simulink model "PID_AutoTuning_tester"  (R2024b)
settings: Solver=FixedStepDiscrete  StartTime=0.0  StopTime=SimEndTime  FixedStep=TimeStep  RelTol=1e-3
undefined symbols (not defined in the file): ctrl_start_time, deadzone_comp_flag, deadzone_comp_val, I_gain_init, P_gain_init, TimeStep
libraries: slctrl_autotuning x1, slpidlib x1, SignalEditorBlockLib x1
settings Model: DataDictionary=system_data.sldd  Creator=tshintai  LastModifiedBy=tshintai
settings SolverCC: AlgebraicLoopSolver=TrustRegion
settings DataIOCC: SaveOutput=off  SaveTime=off
settings OptimizationCC: ReuseModelBlockBuffer=off
settings DebuggingCC: UnconnectedInputMsg=warning  UnconnectedOutputMsg=warning  UnconnectedLineMsg=warning
settings ModelReferenceCC: EnableRefExpFcnMdlSchedulingChecks=on
settings RTWCC: GPUComputeCapability=3.5  DLArmComputeVersion=19.05

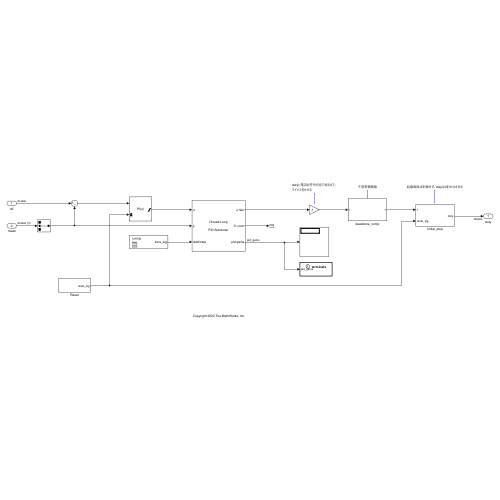
[thumbnail: Simulink's stored preview of the top-level diagram]
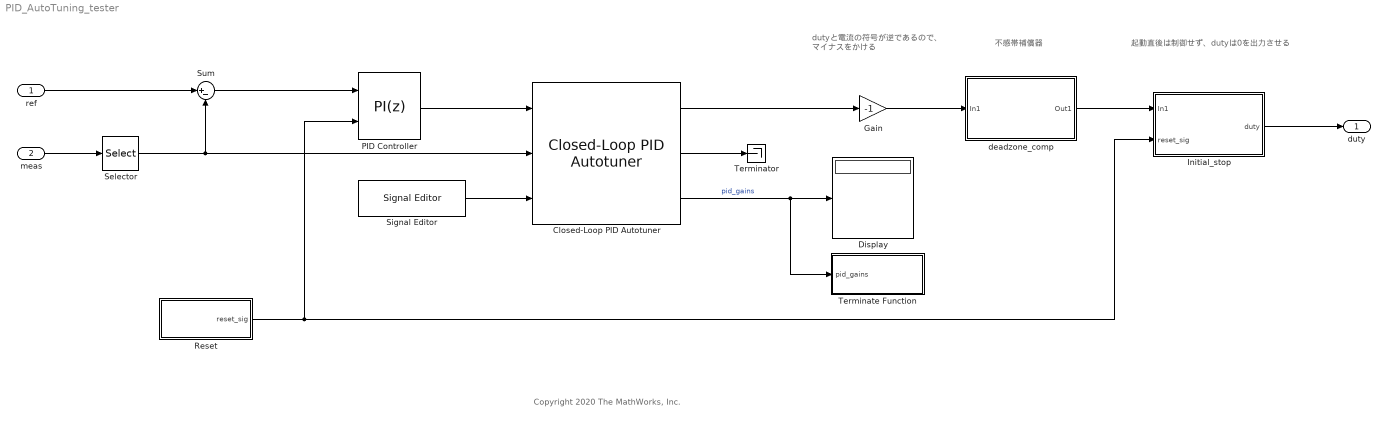
== system PID_AutoTuning_tester ==
  note: Copyright 2020 The MathWorks, Inc.
  note: dutyと電流の符号が逆であるので、
      | マイナスをかける
  note: 起動直後は制御せず、dutyは0を出力させる
  note: 不感帯補償器
  ref : Inport  OutDataTypeStr=double  PortDimensions=1  SampleTime=[0.0001,0]
  meas : Inport  Port=2  OutDataTypeStr=double  PortDimensions=3  SampleTime=[0.0001,0]
  Closed-Loop PID Autotuner : slctrl_autotuning/Closed-Loop PID Autotuner  PIDType=PI  PIDForm=Parallel  TimeDomain=discrete-time  DiscreteTs=TimeStep  TuningTs=0.2  UseTuningTs=off  IntegratorFormula=Forward Euler  FilterFormula=Forward Euler  ContinuousTs=0.02  Bandwidth=2000  UseExternalWC=off  TargetPM=60  UseExternalPM=off  UseExternalAchievedPM=off  ExperimentMode=Superposition  PlantType=Integrating  PlantSign=Positive  AmpSine=0.05  UseExternalAmpSine=off  UseExternalFRD=off  UseExternalU0=off  UseCompanion=off  NotDeployTuningModule=off  UsePLCCoder=off  OutputMode=control action + perturbation  BlockDataType=double  UseConnectedPID=on  blockpath=[]  tunedP=0  tunedI=0  tunedD=0  tunedN=100  tunedPM=0  EstimationWindowSize=3  UseExternalTuningParams=off  SingleMultiRateVariant=SingleSamplingRate  NumEstimationPeriods=4  NumSettlingPeriods=2  NumOfPRBSPeriod=1  PRBSSignalOrder=12  ExperimentModeVariant=VariantSuperimposed  OutputChoice=VariantCandD  ConvergenceCalcVariant=ConvSuperpositionPRBSVariant
  Display : Display
  Gain : Gain  Gain=-1
  Initial_stop : Subsystem
  PID Controller : slpidlib/PID Controller  Controller=PI  Form=Parallel  TimeDomain=Discrete-time  UseExternalTs=off  SampleTime=-1  IntegratorMethod=Forward Euler  FilterMethod=Forward Euler  ControllerParametersSource=internal  P=P_gain_init  I=I_gain_init  UseKiTs=off  D=0  UseExternalDerivativeSource=off  N=100  UseFilter=on  TunerSelectOption=Transfer Function Based (PID Tuner App)  InitialConditionSource=internal  InitialConditionForIntegrator=0  InitialConditionForFilter=0  DifferentiatorICPrevScaledInput=0  ExternalReset=level  TrackingMode=off  Kt=1  LimitOutput=on  SatLimitsSource=internal  UpperSaturationLimit=0.7  LowerSaturationLimit=-0.7  LinearizeAsGain=on  AntiWindupMode=clamping  Kb=1  LimitIntegrator=off  UpperIntegratorSaturationLimit=inf  LowerIntegratorSaturationLimit=-inf  POutMin=[]  POutMax=[]  IOutMin=[]  IOutMax=[]  DOutMin=[]  DOutMax=[]  NOutMin=[]  NOutMax=[]  SumOutMin=[]  SumOutMax=[]  SaturationOutMin=[]  SaturationOutMax=[]  PParamMin=[]  PParamMax=[]  IParamMin=[]  IParamMax=[]  DParamMin=[]  DParamMax=[]  NParamMin=[]  NParamMax=[]  KbParamMin=[]  KbParamMax=[]  KtParamMin=[]  KtParamMax=[]  KbOutMin=[]  KbOutMax=[]  KtOutMin=[]  KtOutMax=[]  IntegratorOutMin=[]  IntegratorOutMax=[]  FilterOutMin=[]  FilterOutMax=[]  SumI1OutMin=[]  SumI1OutMax=[]  SumI2OutMin=[]  SumI2OutMax=[]  SumI3OutMin=[]  SumI3OutMax=[]  SumI4OutMin=[]  SumI4OutMax=[]  SumDOutMin=[]  SumDOutMax=[]  DifferentiatorOutMin=[]  DifferentiatorOutMax=[]  FilterDiffOutCoefMin=[]  FilterDiffOutCoefMax=[]  ReciprocalOutMin=[]  ReciprocalOutMax=[]  SumDenOutMin=[]  SumDenOutMax=[]  SumNumOutMin=[]  SumNumOutMax=[]  DivideOutMin=[]  DivideOutMax=[]  UdiffTsProdOutMin=[]  UdiffTsProdOutMax=[]  NTsProdOutMin=[]  NTsProdOutMax=[]  UintegralTsProdOutMin=[]  UintegralTsProdOutMax=[]  UngainTsProdOutMin=[]  UngainTsProdOutMax=[]  ClampingZeroOutDataTypeStr=Inherit: Inherit via back propagation  ClampingZeroOutMin=[]  ClampingZeroOutMax=[]  FilterDenConstantOutDataTypeStr=Inherit: Inherit via back propagation  FilterDenConstantOutMin=[]  FilterDenConstantOutMax=[]  PCopyOutDataTypeStr=Inherit: Inherit via back propagation  PCopyOutMin=[]  PCopyOutMax=[]  NCopyOutDataTypeStr=Inherit: Inherit via back propagation  NCopyOutMin=[]  NCopyOutMax=[]  IntegratorContinuousStateAttributes=''  IntegratorStateMustResolveToSignalObject=off  IntegratorRTWStateStorageClass=Auto  FilterContinuousStateAttributes=''  FilterStateMustResolveToSignalObject=off  FilterRTWStateStorageClass=Auto  ParallelPVariant=InternalParameters  IdealPVariant=Disabled  IVariant=InternalParameters  DVariant=Disabled  IntegratorVariant=Discrete  SatVariant=Enabled  AWVariant=DiscClampingParallel  PCopyVariant=Disabled  TRVariant=Disabled  FdbkBlocksVariant=Forward  IdealPFdbkVariant=Disabled  SatFdbkVariant=Disabled  DerivativeFilterVariant=Disabled  NVariant=Disabled  NCopyVariant=Disabled_SignalSpec  FilterICVariant=Disabled  IntegratorICVariant=InternalICs  ExternalResetVariant=ExternalReset  TRSumVariant=Passthrough  SumFdbkVariant=Disabled  SumVariant=Sum_PI  TsampFilterVariant=InternalTs  TsampNgainVariant=Passthrough  TsampIntegralVariant=Disabled_SignalSpec  ExternalSaturationOutDataTypeStr=Inherit: Same as second input  DerivativeSourceVariant=Disabled  PreIntVariant=InternalPreInt
  Reset : Subsystem
  Selector : Selector  InputPortWidth=3  IndexOptions=Index vector (dialog)  Indices=[2]  OutputSizes=1
  Signal Editor : SignalEditorBlockLib/Signal Editor  FileName=AutoTuner_sig  ActiveScenario=Tuning  ActiveSignal=tune_sig  IsBus=off  OutputBusObjectStr=Bus: BusObject  SampleTime=TimeStep  Interpolate=off  ZeroCross=off  OutputAfterFinalValue=Setting to zero  Unit=inherit  PreserveSignalName=on  ApplySigPropsToAllScenarios=on  ApplySigPropsToAllSignals=off
  Sum : Sum  Inputs=|+-
  Terminate Function : Subsystem  TreatAsAtomicUnit=on
  Terminator : Terminator
  deadzone_comp : Subsystem
  duty : Outport  OutDataTypeStr=double  PortDimensions=1  SampleTime=[0.0001,0]
  wires:
  ref/1 -> Sum/1
  meas/1 -> Selector/1
  Selector/1 -> Closed-Loop PID Autotuner/2, Sum/2
  Sum/1 -> PID Controller/1
  PID Controller/1 -> Closed-Loop PID Autotuner/1
  Gain/1 -> deadzone_comp/1(In1)
  Reset/1(reset_sig) -> PID Controller/2, Initial_stop/2(reset_sig)
  Initial_stop/1(duty) -> duty/1
  deadzone_comp/1(Out1) -> Initial_stop/1(In1)
  Closed-Loop PID Autotuner/1 -> Gain/1
  Closed-Loop PID Autotuner/3 -> Terminate Function/1(pid_gains), Display/1  "pid_gains"
  Signal Editor/1 -> Closed-Loop PID Autotuner/3
  Closed-Loop PID Autotuner/2 -> Terminator/1

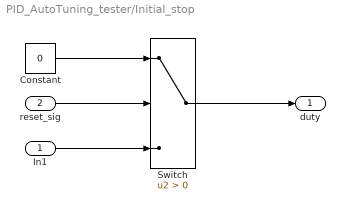
== system PID_AutoTuning_tester/Initial_stop ==
  In1 : Inport
  reset_sig : Inport  Port=2
  Constant : Constant  Value=0
  Switch : Switch  Criteria=u2 > Threshold  SaturateOnIntegerOverflow=off  InputSameDT=off
  duty : Outport
  wires:
  reset_sig/1 -> Switch/2
  Switch/1 -> duty/1
  Constant/1 -> Switch/1
  In1/1 -> Switch/3

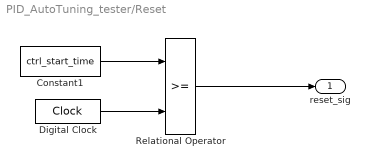
== system PID_AutoTuning_tester/Reset ==
  Constant1 : Constant  Value=ctrl_start_time
  Digital Clock : DigitalClock  SampleTime=TimeStep
  Relational Operator : RelationalOperator  OutDataTypeStr=boolean  RndMeth=Simplest  InputSameDT=off
  reset_sig : Outport
  wires:
  Relational Operator/1 -> reset_sig/1
  Digital Clock/1 -> Relational Operator/2
  Constant1/1 -> Relational Operator/1

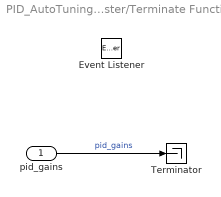
== system PID_AutoTuning_tester/Terminate Function ==
  pid_gains : Inport
  Event Listener : EventListener  DisableCoverage=on  EventType=Terminate  EventName=reset
  Terminator : Terminator
  wires:
  pid_gains/1 -> Terminator/1  "pid_gains"

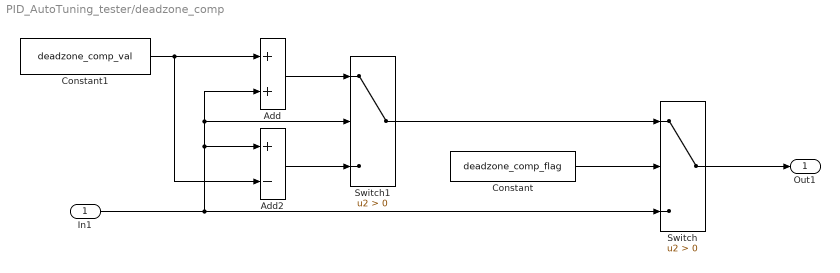
== system PID_AutoTuning_tester/deadzone_comp ==
  In1 : Inport
  Add : Sum
  Add2 : Sum  Inputs=+-
  Constant : Constant  Value=deadzone_comp_flag
  Constant1 : Constant  Value=deadzone_comp_val
  Switch : Switch  Criteria=u2 > Threshold  SaturateOnIntegerOverflow=off  InputSameDT=off
  Switch1 : Switch  Criteria=u2 > Threshold  SaturateOnIntegerOverflow=off  InputSameDT=off
  Out1 : Outport
  wires:
  Switch/1 -> Out1/1
  In1/1 -> Add/2, Switch1/2, Add2/1, Switch/3
  Constant/1 -> Switch/2
  Add/1 -> Switch1/1
  Constant1/1 -> Add2/2, Add/1
  Add2/1 -> Switch1/3
  Switch1/1 -> Switch/1
